simulink model "PMSMSC_FOC1_"  (R2021a)
settings: Solver=FixedStepDiscrete  StartTime=0.0  StopTime=25.0  FixedStep=1  RelTol=1e-3
undefined symbols (not defined in the file): DWORK0, DWORK1, DWORK2, sigbuilder_block, solver_time, speed_ki, speed_kp, Ts, Vd_ki, Vd_kp, Vdc, Vq_ki, Vq_kp
libraries: simulink x1
settings Model: DataDictionary=PMSMSC_FOC_datadictionary.sldd  Creator=comp  LastModifiedBy=LENOVO
settings SolverCC: AlgebraicLoopSolver=TrustRegion
settings OptimizationCC: DefaultParameterBehavior=Inlined  EnhancedBackFolding=on  PassReuseOutputArgsAs=Individual arguments  ZeroExternalMemoryAtStartup=off  ZeroInternalMemoryAtStartup=off  OptimizeBlockOrder=speed  DifferentSizesBufferReuse=on  OptimizationCustomize=off  EfficientTunableParamExpr=on
settings DebuggingCC: SignalInfNanChecking=error  ParameterPrecisionLossMsg=none  ParameterTunabilityLossMsg=error  UniqueDataStoreMsg=warning  SFMachineParentedDataDiag=warning
settings SFSimCC: MATLABDynamicMemAlloc=off  CustomCodeUndefinedFunction=UseInterfaceOnly
settings RTWCC: SystemTargetFile=ert.tlc  GenCodeOnly=on  TemplateMakefile=ert_default_tmf  GenerateReport=on  IncludeHyperlinkInReport=on  LaunchReport=on  GenerateTraceInfo=on  GenerateTraceReport=on  GenerateTraceReportSl=on
settings CodeAppCC: ForceParamTrailComments=on  IgnoreCustomStorageClasses=off  OperatorAnnotations=on  SimulinkDataObjDesc=on  SFDataObjDesc=on  InsertBlockDesc=on
settings ERTTargetCC: TargetLangStandard=C99 (ISO)  GenerateSampleERTMain=on  InlinedParameterPlacement=NonHierarchical  ERTCustomFileTemplate=example_file_process.tlc
settings ConfigComp: CovMetricSettings=dzw

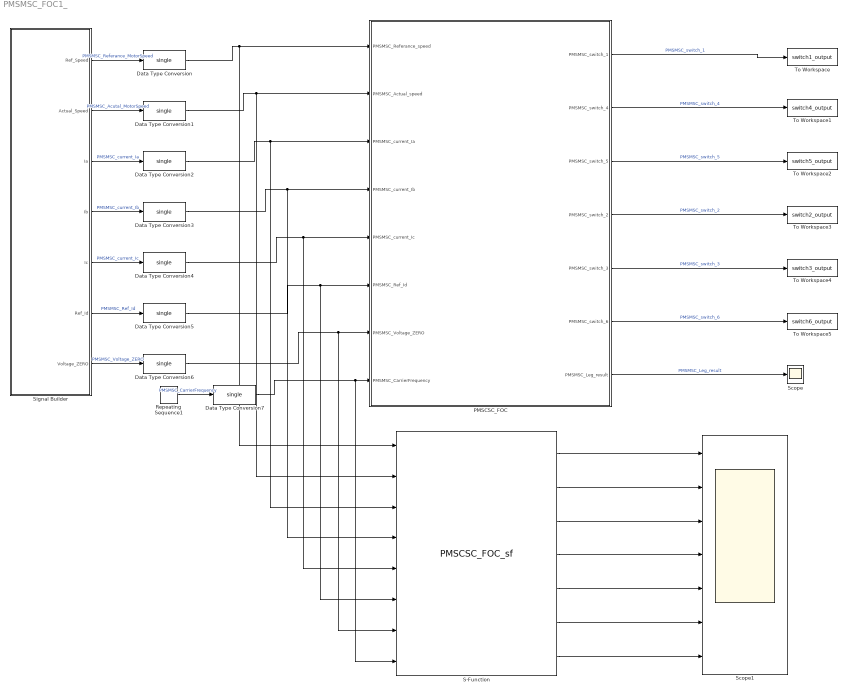
== system PMSMSC_FOC1_ ==
  Data Type Conversion{,1..7} (8 alike) : DataTypeConversion  OutDataTypeStr=single
  PMSCSC_FOC : Subsystem  TreatAsAtomicUnit=on
  Repeating Sequence1 : simulink/Sources/Repeating Sequence  rep_seq_t=[0 1]*[1/3000]  rep_seq_y=[0 0.02]
  S-Function : S-Function  FunctionName=PMSCSC_FOC_sf  SFunctionDeploymentMode=off  EnableBusSupport=off  SFcnStateName=DWORK0,DWORK1,DWORK2
      settings: SFcnIsStateOwnerBlock=on
  Scope : Scope
  Scope1 : Scope  NumInputPorts=7
  Signal Builder : Subsystem  Tag=STV Subsys  LoadFcn=sigbuilder_block('load');  StartFcn=sigbuilder_block('start');  StopFcn=sigbuilder_block('stop');  ClipboardFcn=sigbuilder_block('clipboard');  mask(Sigbuilder block){tuvar=[0:10]}
      mask help: Simulink:masks:SigbuilderBlock_MD
      mask init:
      | if ~strcmp(get_param(bdroot(gcbh),'SimulationStatus'),'stopped') tuvar = sigbuilder_block('maskInit'); end
      settings: CopyFcn=sigbuilder_block('copy');  DeleteFcn=sigbuilder_block('delete');  ModelCloseFcn=sigbuilder_block('modelClose');  PreSaveFcn=sigbuilder_block('preSave');  PauseFcn=sigbuilder_block('pause');  ContinueFcn=sigbuilder_block('continue');  NameChangeFcn=sigbuilder_block('namechange');  OpenFcn=sigbuilder_block('open',[6 30 1012.5 447.75 ]);  CloseFcn=sigbuilder_block('close');
      mask Display: plot(0, 0, 100, 100,[2, 2, 32, 32, 2], [68, 8, 8, 68, 68],[32, 2], [38, 38], [32, 19, 2],[53, 60, 44], [32, 17, 17, 2],[16, 16, 31, 31]);txt = getActiveGroup(gcbh);text(2, 100, txt,'verticalAlignment', 'top');
  To Workspace : ToWorkspace  VariableName=switch1_output  SaveFormat=Timeseries  SampleTime=-1
  To Workspace1 : ToWorkspace  VariableName=switch4_output  SaveFormat=Timeseries  SampleTime=-1
  To Workspace2 : ToWorkspace  VariableName=switch5_output  SaveFormat=Timeseries  SampleTime=-1
  To Workspace3 : ToWorkspace  VariableName=switch2_output  SaveFormat=Timeseries  SampleTime=-1
  To Workspace4 : ToWorkspace  VariableName=switch3_output  SaveFormat=Timeseries  SampleTime=-1
  To Workspace5 : ToWorkspace  VariableName=switch6_output  SaveFormat=Timeseries  SampleTime=-1
  wires:
  Signal Builder/3(Ia) -> Data Type Conversion2/1  "PMSMSC_current_Ia"
  PMSCSC_FOC/1(PMSMSC_switch_1) -> To Workspace/1  "PMSMSC_switch_1"
  PMSCSC_FOC/2(PMSMSC_switch_4) -> To Workspace1/1  "PMSMSC_switch_4"
  PMSCSC_FOC/3(PMSMSC_switch_5) -> To Workspace2/1  "PMSMSC_switch_5"
  PMSCSC_FOC/4(PMSMSC_switch_2) -> To Workspace3/1  "PMSMSC_switch_2"
  PMSCSC_FOC/6(PMSMSC_switch_6) -> To Workspace5/1  "PMSMSC_switch_6"
  PMSCSC_FOC/5(PMSMSC_switch_3) -> To Workspace4/1  "PMSMSC_switch_3"
  PMSCSC_FOC/7(PMSMSC_Leg_result) -> Scope/1  "PMSMSC_Leg_result"
  Repeating Sequence1/1 -> Data Type Conversion7/1  "PMSMSC_CarrierFrequency"
  Signal Builder/1(Ref_Speed) -> Data Type Conversion/1  "PMSMSC_Referance_MotorSpeed"
  Signal Builder/4(Ib) -> Data Type Conversion3/1  "PMSMSC_current_Ib"
  Signal Builder/7(Voltage_ZERO) -> Data Type Conversion6/1  "PMSMSC_Voltage_ZERO"
  Signal Builder/2(Actual_Speed) -> Data Type Conversion1/1  "PMSMSC_Acutal_MotorSpeed"
  Signal Builder/6(Ref_Id) -> Data Type Conversion5/1  "PMSMSC_Ref_Id"
  Signal Builder/5(Ic) -> Data Type Conversion4/1  "PMSMSC_current_Ic"
  Data Type Conversion/1 -> S-Function/1, PMSCSC_FOC/1(PMSMSC_Referance_speed)
  Data Type Conversion1/1 -> PMSCSC_FOC/2(PMSMSC_Actual_speed), S-Function/2
  Data Type Conversion2/1 -> PMSCSC_FOC/3(PMSMSC_current_Ia), S-Function/3
  Data Type Conversion3/1 -> PMSCSC_FOC/4(PMSMSC_current_Ib), S-Function/4
  Data Type Conversion4/1 -> PMSCSC_FOC/5(PMSMSC_current_Ic), S-Function/5
  Data Type Conversion5/1 -> PMSCSC_FOC/6(PMSMSC_Ref_Id), S-Function/6
  Data Type Conversion6/1 -> PMSCSC_FOC/7(PMSMSC_Voltage_ZERO), S-Function/7
  Data Type Conversion7/1 -> PMSCSC_FOC/8(PMSMSC_CarrierFrequency), S-Function/8
  S-Function/1 -> Scope1/1
  S-Function/2 -> Scope1/2
  S-Function/3 -> Scope1/3
  S-Function/4 -> Scope1/4
  S-Function/5 -> Scope1/5
  S-Function/6 -> Scope1/6
  S-Function/7 -> Scope1/7

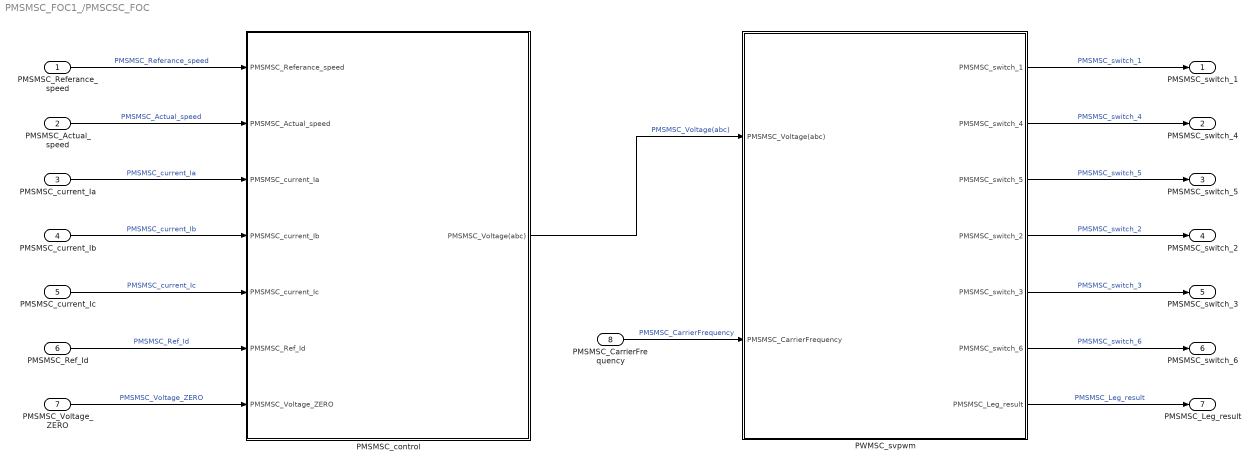
== system PMSMSC_FOC1_/PMSCSC_FOC ==
  PMSMSC_Referance_speed : Inport  OutDataTypeStr=single
  PMSMSC_Actual_speed : Inport  Port=2  OutDataTypeStr=single
  PMSMSC_current_Ia : Inport  Port=3  OutDataTypeStr=single
  PMSMSC_current_Ib : Inport  Port=4  OutDataTypeStr=single
  PMSMSC_current_Ic : Inport  Port=5  OutDataTypeStr=single
  PMSMSC_Ref_Id : Inport  Port=6  OutDataTypeStr=single
  PMSMSC_Voltage_ZERO : Inport  Port=7  OutDataTypeStr=single
  PMSMSC_CarrierFrequency : Inport  Port=8  OutDataTypeStr=single
  PMSMSC_control : Subsystem  TreatAsAtomicUnit=on
  PWMSC_svpwm : Subsystem  TreatAsAtomicUnit=on
  PMSMSC_switch_1 : Outport  OutDataTypeStr=single  VectorParamsAs1DForOutWhenUnconnected=off
  PMSMSC_switch_4 : Outport  Port=2  OutDataTypeStr=single  VectorParamsAs1DForOutWhenUnconnected=off
  PMSMSC_switch_5 : Outport  Port=3  OutDataTypeStr=single  VectorParamsAs1DForOutWhenUnconnected=off
  PMSMSC_switch_2 : Outport  Port=4  OutDataTypeStr=single  VectorParamsAs1DForOutWhenUnconnected=off
  PMSMSC_switch_3 : Outport  Port=5  OutDataTypeStr=single  VectorParamsAs1DForOutWhenUnconnected=off
  PMSMSC_switch_6 : Outport  Port=6  OutDataTypeStr=single  VectorParamsAs1DForOutWhenUnconnected=off
  PMSMSC_Leg_result : Outport  Port=7  OutDataTypeStr=single  VectorParamsAs1DForOutWhenUnconnected=off
  wires:
  PMSMSC_current_Ic/1 -> PMSMSC_control/5("PMSMSC_current_Ic ")  "PMSMSC_current_Ic"
  PMSMSC_Actual_speed/1 -> PMSMSC_control/2(PMSMSC_Actual_speed)  "PMSMSC_Actual_speed"
  PWMSC_svpwm/1(PMSMSC_switch_1) -> PMSMSC_switch_1/1  "PMSMSC_switch_1"
  PWMSC_svpwm/2(PMSMSC_switch_4) -> PMSMSC_switch_4/1  "PMSMSC_switch_4"
  PWMSC_svpwm/5(PMSMSC_switch_3) -> PMSMSC_switch_3/1  "PMSMSC_switch_3"
  PMSMSC_control/1(PMSMSC_Voltage(abc)) -> PWMSC_svpwm/1(PMSMSC_Voltage(abc))  "PMSMSC_Voltage(abc)"
  PWMSC_svpwm/3(PMSMSC_switch_5) -> PMSMSC_switch_5/1  "PMSMSC_switch_5"
  PWMSC_svpwm/4(PMSMSC_switch_2) -> PMSMSC_switch_2/1  "PMSMSC_switch_2"
  PMSMSC_Referance_speed/1 -> PMSMSC_control/1(PMSMSC_Referance_speed)  "PMSMSC_Referance_speed"
  PMSMSC_current_Ia/1 -> PMSMSC_control/3("PMSMSC_current_Ia ")  "PMSMSC_current_Ia"
  PMSMSC_current_Ib/1 -> PMSMSC_control/4("PMSMSC_current_Ib ")  "PMSMSC_current_Ib"
  PWMSC_svpwm/6(PMSMSC_switch_6) -> PMSMSC_switch_6/1  "PMSMSC_switch_6"
  PMSMSC_Ref_Id/1 -> PMSMSC_control/6("PMSMSC_Ref_Id ")  "PMSMSC_Ref_Id"
  PMSMSC_Voltage_ZERO/1 -> PMSMSC_control/7("PMSMSC_Voltage_ZERO ")  "PMSMSC_Voltage_ZERO"
  PWMSC_svpwm/7(PMSMSC_Leg_result) -> PMSMSC_Leg_result/1  "PMSMSC_Leg_result"
  PMSMSC_CarrierFrequency/1 -> PWMSC_svpwm/2(PMSMSC_CarrierFrequency)  "PMSMSC_CarrierFrequency"

== system PMSMSC_FOC1_/Signal Builder ==
  Demux : Demux  Tag=STV Demux  Outputs=7
      settings: DisplayOption=none
  FromWs : FromWorkspace  Tag=STV FromWs  VariableName=tuvar
      SigBuilderData=|
      | common.afterFinalStr = 'Extrapolate'
      | common.sampleTime = 0
      | dataSet.timeRange = [0 20]
      | dataSet.name = 'Sheet1'
      | sbobj.Name = 'Signal Builder'
      | sbobj.Groups.Name = 'Sheet1'
      | sbobj.Groups.Signals(1).Name = 'Ref_Speed'
      | sbobj.Groups.Signals(1).XData = [0 1 2 3 4 5 6 7 8 9 10 11 12 13 14 15 16 17 18 19 20]
      | sbobj.Groups.Signals(1).YData = [1200 1200 1200 1200 1200 1200 1200 1200 1200 1200 1200 1200 1200 1200 1200 1200 1200 1200 1200 1200 1200]
      | sbobj.Groups.Signals(2).Name = 'Actual_Speed'
      | sbobj.Groups.Signals(2).XData = [0 1 2 3 4 5 6 7 8 9 10 11 12 13 14 15 16 17 18 19 20]
      | sbobj.Groups.Signals(2).YData = [0 200 400 600 800 1000 1200 1400 1100 1150 1200 1250 1200 1280 1200 1270 1200 1260 1250 1200 1200]
      | sbobj.Groups.Signals(3).Name = 'Ia'
      | sbobj.Groups.Signals(3).XData = [0 1 2 3 4 5 6 7 8 9 10 11 12 13 14 15 16 17 18 19 20]
      | sbobj.Groups.Signals(3).YData = [0 10 20 30 40 50 60 50 60 60 60 60 60 60 60 60 60 60 60 60 60]
      | sbobj.Groups.Signals(4).Name = 'Ib'
      | sbobj.Groups.Signals(4).XData = [0 1 2 3 4 5 6 7 8 9 10 11 12 13 14 15 16 17 18 19 20]
      | sbobj.Groups.Signals(4).YData = [0 10 20 30 40 50 60 50 60 60 60 60 60 60 60 60 60 60 60 60 60]
      | sbobj.Groups.Signals(5).Name = 'Ic'
      | sbobj.Groups.Signals(5).XData = [0 1 2 3 4 5 6 7 8 9 10 11 12 13 14 15 16 17 18 19 20]
      | sbobj.Groups.Signals(5).YData = [0 10 20 30 40 50 60 50 60 60 60 60 60 60 60 60 60 60 60 60 60]
      | sbobj.Groups.Signals(6).Name = 'Ref_Id'
      | sbobj.Groups.Signals(6).XData = [0 1 2 3 4 5 6 7 8 9 10 11 12 13 14 15 16 17 18 19 20]
      | sbobj.Groups.Signals(6).YData = [0 0 0 0 0 0 0 0 0 0 0 0 0 0 0 0 0 0 0 0 0]
      | sbobj.Groups.Signals(7).Name = 'Voltage_ZERO'
      | sbobj.Groups.Signals(7).XData = [0 1 2 3 4 5 6 7 8 9 10 11 12 13 14 15 16 17 18 19 20]
      | sbobj.Groups.Signals(7).YData = [0 0 0 0 0 0 0 0 0 0 0 0 0 0 0 0 0 0 0 0 0]
      | sbobj.Groups.TimeRange = [0 20]
  Ref_Speed : Outport  Tag=STV Outport
  Actual_Speed : Outport  Tag=STV Outport  Port=2
  Ia : Outport  Tag=STV Outport  Port=3
  Ib : Outport  Tag=STV Outport  Port=4
  Ic : Outport  Tag=STV Outport  Port=5
  Ref_Id : Outport  Tag=STV Outport  Port=6
  Voltage_ZERO : Outport  Tag=STV Outport  Port=7
  wires:
  Demux/1 -> Ref_Speed/1
  FromWs/1 -> Demux/1
  Demux/2 -> Actual_Speed/1
  Demux/3 -> Ia/1
  Demux/4 -> Ib/1
  Demux/5 -> Ic/1
  Demux/6 -> Ref_Id/1
  Demux/7 -> Voltage_ZERO/1

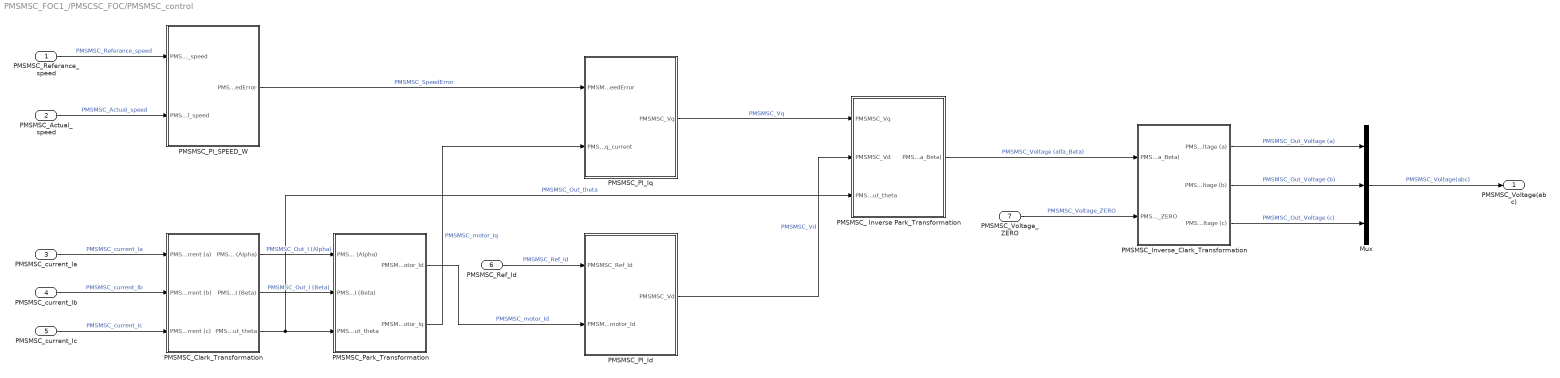
== system PMSMSC_FOC1_/PMSCSC_FOC/PMSMSC_control ==
  PMSMSC_Referance_speed : Inport  OutDataTypeStr=single
  PMSMSC_Actual_speed : Inport  Port=2  OutDataTypeStr=single
  "PMSMSC_current_Ia " : Inport  Port=3  OutDataTypeStr=single
  "PMSMSC_current_Ib " : Inport  Port=4  OutDataTypeStr=single
  "PMSMSC_current_Ic " : Inport  Port=5  OutDataTypeStr=single
  "PMSMSC_Ref_Id " : Inport  Port=6  OutDataTypeStr=single
  "PMSMSC_Voltage_ZERO " : Inport  Port=7  OutDataTypeStr=single
  Mux : Mux  Inputs=3
  PMSMSC_ Inverse Park_Transformation : Subsystem  TreatAsAtomicUnit=on
  "PMSMSC_Clark_Transformation " : Subsystem  TreatAsAtomicUnit=on
  PMSMSC_Inverse_Clark_Transformation : Subsystem  TreatAsAtomicUnit=on
  "PMSMSC_PI_Id " : Subsystem  TreatAsAtomicUnit=on
  "PMSMSC_PI_Iq " : Subsystem  TreatAsAtomicUnit=on
  "PMSMSC_PI_SPEED_W " : Subsystem  TreatAsAtomicUnit=on
  "PMSMSC_Park_Transformation " : Subsystem  TreatAsAtomicUnit=on
  PMSMSC_Voltage(abc) : Outport  OutDataTypeStr=single  VectorParamsAs1DForOutWhenUnconnected=off
  wires:
  PMSMSC_Inverse_Clark_Transformation/3("PMSMSC_Out_Voltage (c) ") -> Mux/3  "PMSMSC_Out_Voltage (c)"
  PMSMSC_Inverse_Clark_Transformation/1("PMSMSC_Out_Voltage (a) ") -> Mux/1  "PMSMSC_Out_Voltage (a)"
  PMSMSC_Actual_speed/1 -> "PMSMSC_PI_SPEED_W "/2(PMSMSC_Actual_speed)  "PMSMSC_Actual_speed"
  PMSMSC_Referance_speed/1 -> "PMSMSC_PI_SPEED_W "/1(PMSMSC_Referance_speed)  "PMSMSC_Referance_speed"
  "PMSMSC_Park_Transformation "/2(PMSMSC_motor_Iq) -> "PMSMSC_PI_Iq "/2(PMSMSC_Iq_current)  "PMSMSC_motor_Iq"
  "PMSMSC_Park_Transformation "/1("PMSMSC_motor_Id ") -> "PMSMSC_PI_Id "/2("PMSMSC_motor_Id ")  "PMSMSC_motor_Id"
  "PMSMSC_Ref_Id "/1 -> "PMSMSC_PI_Id "/1("PMSMSC_Ref_Id ")  "PMSMSC_Ref_Id"
  "PMSMSC_Clark_Transformation "/1(PMSMSC_Out_I (Alpha)) -> "PMSMSC_Park_Transformation "/1("PMSMSC_Out_I (Alpha) ")  "PMSMSC_Out_I (Alpha)"
  "PMSMSC_Clark_Transformation "/2(PMSMSC_Out_I (Beta)) -> "PMSMSC_Park_Transformation "/2("PMSMSC_Out_I (Beta) ")  "PMSMSC_Out_I (Beta)"
  "PMSMSC_PI_SPEED_W "/1(PMSMSC_SpeedError) -> "PMSMSC_PI_Iq "/1(PMSMSC_SpeedError)  "PMSMSC_SpeedError"
  "PMSMSC_PI_Id "/1("PMSMSC_Vd ") -> PMSMSC_ Inverse Park_Transformation/2("PMSMSC_Vd ")  "PMSMSC_Vd"
  "PMSMSC_PI_Iq "/1(PMSMSC_Vq) -> PMSMSC_ Inverse Park_Transformation/1("PMSMSC_Vq ")  "PMSMSC_Vq"
  "PMSMSC_Clark_Transformation "/3(PMSMSC_Out_theta) -> PMSMSC_ Inverse Park_Transformation/3("PMSMSC_Out_theta "), "PMSMSC_Park_Transformation "/3("PMSMSC_Out_theta ")  "PMSMSC_Out_theta"
  "PMSMSC_current_Ia "/1 -> "PMSMSC_Clark_Transformation "/1("PMSMSC_Inv_Out_Current (a) ")  "PMSMSC_current_Ia"
  "PMSMSC_current_Ib "/1 -> "PMSMSC_Clark_Transformation "/2("PMSMSC_Inv_Out_Current (b) ")  "PMSMSC_current_Ib"
  "PMSMSC_current_Ic "/1 -> "PMSMSC_Clark_Transformation "/3("PMSMSC_Inv_Out_Current (c) ")  "PMSMSC_current_Ic"
  Mux/1 -> PMSMSC_Voltage(abc)/1  "PMSMSC_Voltage(abc)"
  PMSMSC_Inverse_Clark_Transformation/2("PMSMSC_Out_Voltage (b) ") -> Mux/2  "PMSMSC_Out_Voltage (b)"
  PMSMSC_ Inverse Park_Transformation/1("PMSMSC_Voltage (alfa_Beta) ") -> PMSMSC_Inverse_Clark_Transformation/1(PMSMSC_Voltage (alfa_Beta))  "PMSMSC_Voltage (alfa_Beta)"
  "PMSMSC_Voltage_ZERO "/1 -> PMSMSC_Inverse_Clark_Transformation/2(PMSMSC_Voltage_ZERO)  "PMSMSC_Voltage_ZERO"

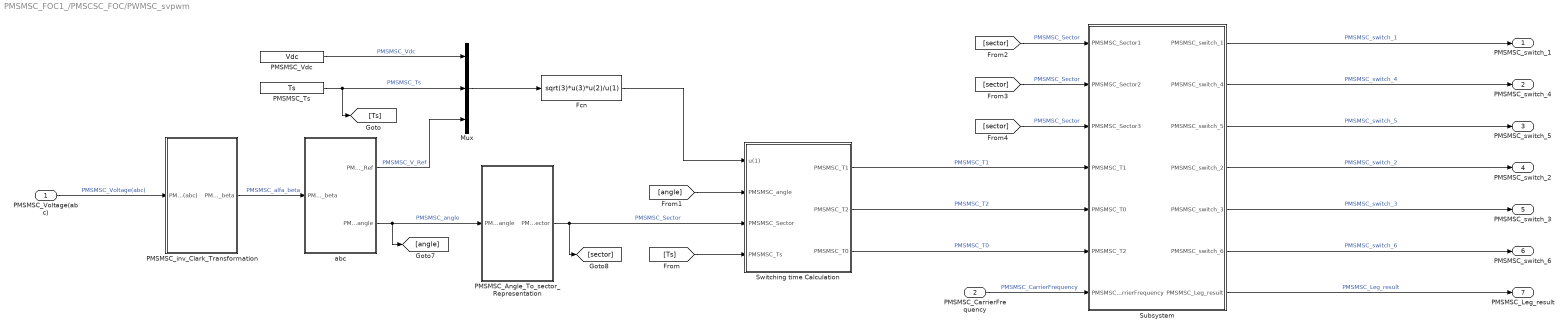
== system PMSMSC_FOC1_/PMSCSC_FOC/PWMSC_svpwm ==
  PMSMSC_Voltage(abc) : Inport  OutDataTypeStr=single
  PMSMSC_CarrierFrequency : Inport  Port=2  OutDataTypeStr=single
  Fcn : Fcn  Expr=sqrt(3)*u(3)*u(2)/u(1)
  Mux : Mux  Inputs=3
  PMSMSC_Angle_To_sector_Representation : Subsystem  TreatAsAtomicUnit=on
  PMSMSC_Ts : Constant  Value=Ts
  PMSMSC_Vdc : Constant  Value=Vdc
  PMSMSC_inv_Clark_Transformation : Subsystem  TreatAsAtomicUnit=on
  Subsystem : Subsystem  TreatAsAtomicUnit=on
  Switching time Calculation : Subsystem  TreatAsAtomicUnit=on
  abc : Subsystem  TreatAsAtomicUnit=on
  PMSMSC_switch_1 : Outport  OutDataTypeStr=single  VectorParamsAs1DForOutWhenUnconnected=off
  PMSMSC_switch_4 : Outport  Port=2  OutDataTypeStr=single  VectorParamsAs1DForOutWhenUnconnected=off
  PMSMSC_switch_5 : Outport  Port=3  OutDataTypeStr=single  VectorParamsAs1DForOutWhenUnconnected=off
  PMSMSC_switch_2 : Outport  Port=4  OutDataTypeStr=single  VectorParamsAs1DForOutWhenUnconnected=off
  PMSMSC_switch_3 : Outport  Port=5  OutDataTypeStr=single  VectorParamsAs1DForOutWhenUnconnected=off
  PMSMSC_switch_6 : Outport  Port=6  OutDataTypeStr=single  VectorParamsAs1DForOutWhenUnconnected=off
  PMSMSC_Leg_result : Outport  Port=7  OutDataTypeStr=single  VectorParamsAs1DForOutWhenUnconnected=off
  wires:
  abc/1(PMSMSC_V_Ref) -> Mux/3  "PMSMSC_V_Ref"
  PMSMSC_Vdc/1 -> Mux/1  "PMSMSC_Vdc"
  [Ts] -> Switching time Calculation/4(PMSMSC_Ts)
  [angle] -> Switching time Calculation/2(PMSMSC_angle)
  [sector] -> Subsystem/1(PMSMSC_Sector1)  "PMSMSC_Sector"
  Mux/1 -> Fcn/1
  abc/2("PMSMSC_angle ") -> [angle], PMSMSC_Angle_To_sector_Representation/1(PMSMSC_angle)  "PMSMSC_angle"
  Switching time Calculation/2(PMSMSC_T2) -> Subsystem/5(PMSMSC_T0)  "PMSMSC_T2"
  Subsystem/1(PMSMSC_switch_1) -> PMSMSC_switch_1/1  "PMSMSC_switch_1"
  [sector] -> Subsystem/3(PMSMSC_Sector3)  "PMSMSC_Sector"
  Fcn/1 -> Switching time Calculation/1(u(1))
  PMSMSC_Voltage(abc)/1 -> PMSMSC_inv_Clark_Transformation/1(PMSMSC_Voltage(abc))  "PMSMSC_Voltage(abc)"
  Switching time Calculation/1(PMSMSC_T1) -> Subsystem/4(PMSMSC_T1)  "PMSMSC_T1"
  PMSMSC_Angle_To_sector_Representation/1(PMSMSC_Sector) -> [sector], Switching time Calculation/3(PMSMSC_Sector)  "PMSMSC_Sector"
  PMSMSC_inv_Clark_Transformation/1(PMSMSC_alfa_beta) -> abc/1(PMSMSC_alfa_beta)  "PMSMSC_alfa_beta"
  PMSMSC_Ts/1 -> Mux/2, [Ts]  "PMSMSC_Ts"
  Subsystem/4(PMSMSC_switch_2) -> PMSMSC_switch_2/1  "PMSMSC_switch_2"
  Subsystem/3(PMSMSC_switch_5) -> PMSMSC_switch_5/1  "PMSMSC_switch_5"
  Switching time Calculation/3(PMSMSC_T0) -> Subsystem/6(PMSMSC_T2)  "PMSMSC_T0"
  [sector] -> Subsystem/2(PMSMSC_Sector2)  "PMSMSC_Sector"
  Subsystem/2(PMSMSC_switch_4) -> PMSMSC_switch_4/1  "PMSMSC_switch_4"
  Subsystem/6(PMSMSC_switch_6) -> PMSMSC_switch_6/1  "PMSMSC_switch_6"
  Subsystem/5(PMSMSC_switch_3) -> PMSMSC_switch_3/1  "PMSMSC_switch_3"
  Subsystem/7(PMSMSC_Leg_result) -> PMSMSC_Leg_result/1  "PMSMSC_Leg_result"
  PMSMSC_CarrierFrequency/1 -> Subsystem/7(PMSMSC_CarrierFrequency)  "PMSMSC_CarrierFrequency"

== system PMSMSC_FOC1_/PMSCSC_FOC/PMSMSC_control/PMSMSC_ Inverse Park_Transformation ==
  "PMSMSC_Vq " : Inport  OutDataTypeStr=single
  "PMSMSC_Vd " : Inport  Port=2  OutDataTypeStr=single
  "PMSMSC_Out_theta " : Inport  Port=3  OutDataTypeStr=single
  Mux : Mux  Inputs=3
  Mux1 : Mux  Inputs=2
  current_to_voltage_alfa : Fcn  Expr=u(1)*cos(u(3))-u(2)*sin(u(3))
  current_to_voltage_beta : Fcn  Expr=u(1)*sin(u(3))+u(2)*cos(u(3))
  "PMSMSC_Voltage (alfa_Beta) " : Outport  OutDataTypeStr=single  VectorParamsAs1DForOutWhenUnconnected=off
  wires:
  Mux1/1 -> "PMSMSC_Voltage (alfa_Beta) "/1  "PMSMSC_Voltage (alfa_Beta)"
  Mux/1 -> current_to_voltage_alfa/1, current_to_voltage_beta/1
  current_to_voltage_alfa/1 -> Mux1/1
  "PMSMSC_Vq "/1 -> Mux/1  "PMSMSC_Vq"
  "PMSMSC_Vd "/1 -> Mux/2  "PMSMSC_Vd"
  current_to_voltage_beta/1 -> Mux1/2
  "PMSMSC_Out_theta "/1 -> Mux/3  "PMSMSC_Out_theta"

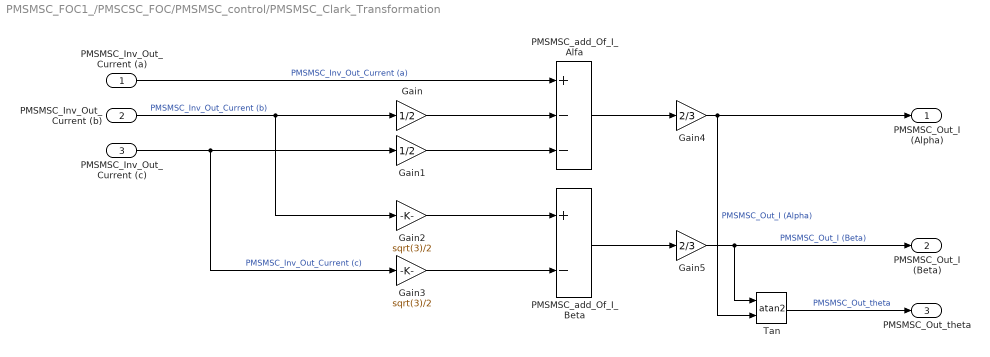
== system PMSMSC_FOC1_/PMSCSC_FOC/PMSMSC_control/PMSMSC_Clark_Transformation  ==
  "PMSMSC_Inv_Out_Current (a) " : Inport  OutDataTypeStr=single
  "PMSMSC_Inv_Out_Current (b) " : Inport  Port=2  OutDataTypeStr=single
  "PMSMSC_Inv_Out_Current (c) " : Inport  Port=3  OutDataTypeStr=single
  Gain : Gain  Gain=1/2  OutDataTypeStr=single
  Gain1 : Gain  Gain=1/2  OutDataTypeStr=single
  Gain2 : Gain  Gain=sqrt(3)/2  OutDataTypeStr=single
  Gain3 : Gain  Gain=sqrt(3)/2  OutDataTypeStr=single
  Gain4 : Gain  Gain=2/3  OutDataTypeStr=single
  Gain5 : Gain  Gain=2/3  OutDataTypeStr=single
  PMSMSC_add_Of_I_Alfa : Sum  Inputs=+--  AccumDataTypeStr=single
  PMSMSC_add_Of_I_Beta : Sum  Inputs=+-  AccumDataTypeStr=single
  Tan : Trigonometry  Operator=atan2
  PMSMSC_Out_I (Alpha) : Outport  OutDataTypeStr=single  VectorParamsAs1DForOutWhenUnconnected=off
  PMSMSC_Out_I (Beta) : Outport  Port=2  OutDataTypeStr=single  VectorParamsAs1DForOutWhenUnconnected=off
  PMSMSC_Out_theta : Outport  Port=3  OutDataTypeStr=single  VectorParamsAs1DForOutWhenUnconnected=off
  wires:
  Gain3/1 -> PMSMSC_add_Of_I_Beta/2
  "PMSMSC_Inv_Out_Current (b) "/1 -> Gain2/1, Gain/1  "PMSMSC_Inv_Out_Current (b)"
  Gain/1 -> PMSMSC_add_Of_I_Alfa/2
  Gain1/1 -> PMSMSC_add_Of_I_Alfa/3
  "PMSMSC_Inv_Out_Current (a) "/1 -> PMSMSC_add_Of_I_Alfa/1  "PMSMSC_Inv_Out_Current (a)"
  "PMSMSC_Inv_Out_Current (c) "/1 -> Gain3/1, Gain1/1  "PMSMSC_Inv_Out_Current (c)"
  PMSMSC_add_Of_I_Alfa/1 -> Gain4/1
  PMSMSC_add_Of_I_Beta/1 -> Gain5/1
  Gain2/1 -> PMSMSC_add_Of_I_Beta/1
  Gain5/1 -> Tan/1, PMSMSC_Out_I (Beta)/1  "PMSMSC_Out_I (Beta)"
  Gain4/1 -> Tan/2, PMSMSC_Out_I (Alpha)/1  "PMSMSC_Out_I (Alpha)"
  Tan/1 -> PMSMSC_Out_theta/1  "PMSMSC_Out_theta"

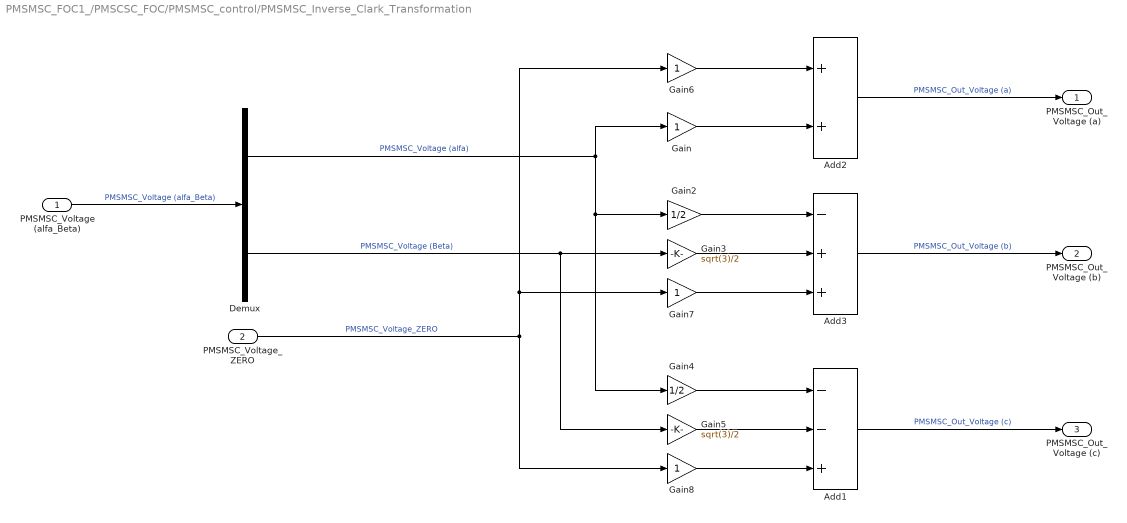
== system PMSMSC_FOC1_/PMSCSC_FOC/PMSMSC_control/PMSMSC_Inverse_Clark_Transformation ==
  PMSMSC_Voltage (alfa_Beta) : Inport  OutDataTypeStr=single
  PMSMSC_Voltage_ZERO : Inport  Port=2  OutDataTypeStr=single
  Add1 : Sum  Inputs=--+  AccumDataTypeStr=single
  Add2 : Sum  AccumDataTypeStr=single
  Add3 : Sum  Inputs=-++  AccumDataTypeStr=single
  Demux : Demux  Outputs=2
  Gain{,6..8} (4 alike) : Gain  OutDataTypeStr=single
  Gain2 : Gain  Gain=1/2  OutDataTypeStr=single
  Gain3 : Gain  Gain=sqrt(3)/2  OutDataTypeStr=single  SaturateOnIntegerOverflow=on
  Gain4 : Gain  Gain=1/2  OutDataTypeStr=single
  Gain5 : Gain  Gain=sqrt(3)/2  OutDataTypeStr=single
  "PMSMSC_Out_Voltage (a) " : Outport  OutDataTypeStr=single  VectorParamsAs1DForOutWhenUnconnected=off
  "PMSMSC_Out_Voltage (b) " : Outport  Port=2  OutDataTypeStr=single  VectorParamsAs1DForOutWhenUnconnected=off
  "PMSMSC_Out_Voltage (c) " : Outport  Port=3  OutDataTypeStr=single  VectorParamsAs1DForOutWhenUnconnected=off
  wires:
  Add3/1 -> "PMSMSC_Out_Voltage (b) "/1  "PMSMSC_Out_Voltage (b)"
  Add2/1 -> "PMSMSC_Out_Voltage (a) "/1  "PMSMSC_Out_Voltage (a)"
  Gain5/1 -> Add1/2
  Gain4/1 -> Add1/1
  Demux/2 -> Gain3/1, Gain5/1  "PMSMSC_Voltage (Beta)"
  Add1/1 -> "PMSMSC_Out_Voltage (c) "/1  "PMSMSC_Out_Voltage (c)"
  PMSMSC_Voltage_ZERO/1 -> Gain6/1, Gain7/1, Gain8/1  "PMSMSC_Voltage_ZERO"
  Demux/1 -> Gain/1, Gain2/1, Gain4/1  "PMSMSC_Voltage (alfa)"
  Gain3/1 -> Add3/2
  Gain8/1 -> Add1/3
  Gain2/1 -> Add3/1
  Gain6/1 -> Add2/1
  Gain/1 -> Add2/2
  Gain7/1 -> Add3/3
  PMSMSC_Voltage (alfa_Beta)/1 -> Demux/1  "PMSMSC_Voltage (alfa_Beta)"

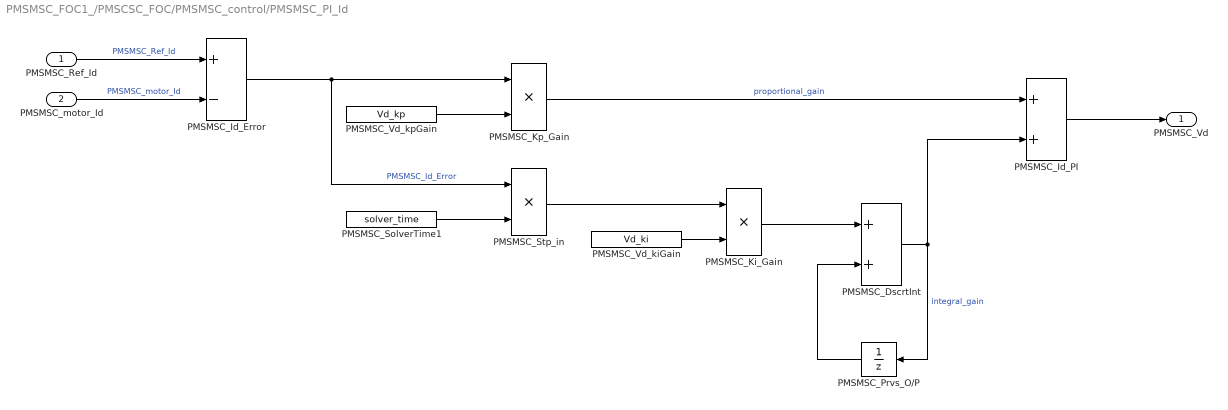
== system PMSMSC_FOC1_/PMSCSC_FOC/PMSMSC_control/PMSMSC_PI_Id  ==
  "PMSMSC_Ref_Id " : Inport  OutDataTypeStr=single
  "PMSMSC_motor_Id " : Inport  Port=2  OutDataTypeStr=single
  "PMSMSC_DscrtInt " : Sum  AccumDataTypeStr=single
  PMSMSC_Id_Error : Sum  Inputs=+-  AccumDataTypeStr=single
  PMSMSC_Id_PI : Sum  AccumDataTypeStr=single
  PMSMSC_Ki_Gain : Product  OutDataTypeStr=single
  PMSMSC_Kp_Gain : Product  OutDataTypeStr=single
  PMSMSC_Prvs_O/P : UnitDelay  SampleTime=-1  HasFrameUpgradeWarning=on
  PMSMSC_SolverTime1 : Constant  Value=solver_time
  "PMSMSC_Stp_in " : Product  OutDataTypeStr=single
  PMSMSC_Vd_kiGain : Constant  Value=Vd_ki
  PMSMSC_Vd_kpGain : Constant  Value=Vd_kp
  "PMSMSC_Vd " : Outport  OutDataTypeStr=single  VectorParamsAs1DForOutWhenUnconnected=off
  wires:
  PMSMSC_Kp_Gain/1 -> PMSMSC_Id_PI/1  "proportional_gain"
  PMSMSC_Vd_kiGain/1 -> PMSMSC_Ki_Gain/2
  PMSMSC_Ki_Gain/1 -> "PMSMSC_DscrtInt "/1
  PMSMSC_Vd_kpGain/1 -> PMSMSC_Kp_Gain/2
  PMSMSC_SolverTime1/1 -> "PMSMSC_Stp_in "/2
  "PMSMSC_motor_Id "/1 -> PMSMSC_Id_Error/2  "PMSMSC_motor_Id"
  PMSMSC_Id_PI/1 -> "PMSMSC_Vd "/1
  PMSMSC_Prvs_O/P/1 -> "PMSMSC_DscrtInt "/2
  PMSMSC_Id_Error/1 -> PMSMSC_Kp_Gain/1, "PMSMSC_Stp_in "/1  "PMSMSC_Id_Error"
  "PMSMSC_DscrtInt "/1 -> PMSMSC_Id_PI/2, PMSMSC_Prvs_O/P/1  "integral_gain"
  "PMSMSC_Ref_Id "/1 -> PMSMSC_Id_Error/1  "PMSMSC_Ref_Id"
  "PMSMSC_Stp_in "/1 -> PMSMSC_Ki_Gain/1

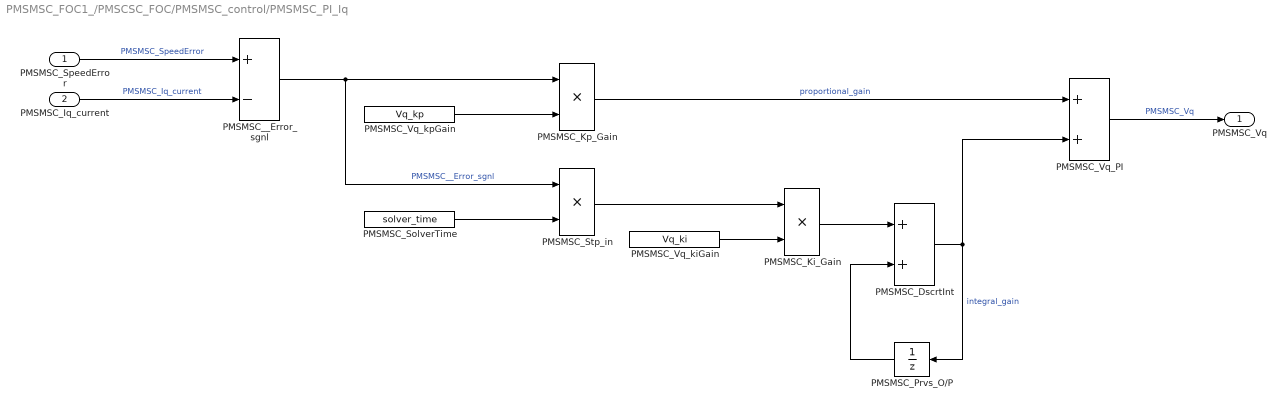
== system PMSMSC_FOC1_/PMSCSC_FOC/PMSMSC_control/PMSMSC_PI_Iq  ==
  PMSMSC_SpeedError : Inport  OutDataTypeStr=single
  PMSMSC_Iq_current : Inport  Port=2  OutDataTypeStr=single
  "PMSMSC_DscrtInt " : Sum  AccumDataTypeStr=single
  PMSMSC_Ki_Gain : Product  OutDataTypeStr=single
  PMSMSC_Kp_Gain : Product  OutDataTypeStr=single
  PMSMSC_Prvs_O/P : UnitDelay  SampleTime=-1  HasFrameUpgradeWarning=on
  PMSMSC_SolverTime : Constant  Value=solver_time
  "PMSMSC_Stp_in " : Product  OutDataTypeStr=single
  PMSMSC_Vq_PI : Sum  AccumDataTypeStr=single
  PMSMSC_Vq_kiGain : Constant  Value=Vq_ki
  PMSMSC_Vq_kpGain : Constant  Value=Vq_kp
  PMSMSC__Error_sgnl : Sum  Inputs=+-  AccumDataTypeStr=single
  PMSMSC_Vq : Outport  OutDataTypeStr=single  VectorParamsAs1DForOutWhenUnconnected=off
  wires:
  "PMSMSC_Stp_in "/1 -> PMSMSC_Ki_Gain/1
  PMSMSC_SpeedError/1 -> PMSMSC__Error_sgnl/1  "PMSMSC_SpeedError"
  "PMSMSC_DscrtInt "/1 -> PMSMSC_Vq_PI/2, PMSMSC_Prvs_O/P/1  "integral_gain"
  PMSMSC__Error_sgnl/1 -> "PMSMSC_Stp_in "/1, PMSMSC_Kp_Gain/1  "PMSMSC__Error_sgnl"
  PMSMSC_Prvs_O/P/1 -> "PMSMSC_DscrtInt "/2
  PMSMSC_Vq_PI/1 -> PMSMSC_Vq/1  "PMSMSC_Vq"
  PMSMSC_Iq_current/1 -> PMSMSC__Error_sgnl/2  "PMSMSC_Iq_current"
  PMSMSC_SolverTime/1 -> "PMSMSC_Stp_in "/2
  PMSMSC_Vq_kpGain/1 -> PMSMSC_Kp_Gain/2
  PMSMSC_Ki_Gain/1 -> "PMSMSC_DscrtInt "/1
  PMSMSC_Vq_kiGain/1 -> PMSMSC_Ki_Gain/2
  PMSMSC_Kp_Gain/1 -> PMSMSC_Vq_PI/1  "proportional_gain"

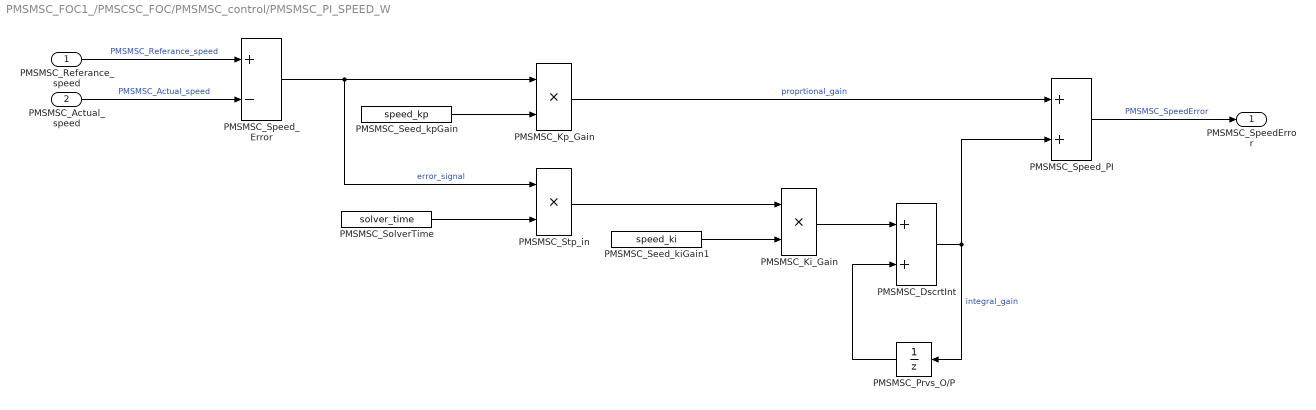
== system PMSMSC_FOC1_/PMSCSC_FOC/PMSMSC_control/PMSMSC_PI_SPEED_W  ==
  PMSMSC_Referance_speed : Inport  OutDataTypeStr=single
  PMSMSC_Actual_speed : Inport  Port=2  OutDataTypeStr=single
  "PMSMSC_DscrtInt " : Sum  AccumDataTypeStr=single
  PMSMSC_Ki_Gain : Product  OutDataTypeStr=single
  PMSMSC_Kp_Gain : Product  OutDataTypeStr=single
  PMSMSC_Prvs_O/P : UnitDelay  SampleTime=-1  HasFrameUpgradeWarning=on
  PMSMSC_Seed_kiGain1 : Constant  Value=speed_ki
  PMSMSC_Seed_kpGain : Constant  Value=speed_kp
  PMSMSC_SolverTime : Constant  Value=solver_time
  PMSMSC_Speed_Error : Sum  Inputs=+-  AccumDataTypeStr=single
  PMSMSC_Speed_PI : Sum  AccumDataTypeStr=single
  "PMSMSC_Stp_in " : Product  OutDataTypeStr=single
  PMSMSC_SpeedError : Outport  OutDataTypeStr=single  VectorParamsAs1DForOutWhenUnconnected=off
  wires:
  PMSMSC_Kp_Gain/1 -> PMSMSC_Speed_PI/1  "proprtional_gain"
  PMSMSC_Seed_kiGain1/1 -> PMSMSC_Ki_Gain/2
  PMSMSC_Ki_Gain/1 -> "PMSMSC_DscrtInt "/1
  PMSMSC_Seed_kpGain/1 -> PMSMSC_Kp_Gain/2
  PMSMSC_SolverTime/1 -> "PMSMSC_Stp_in "/2
  PMSMSC_Speed_PI/1 -> PMSMSC_SpeedError/1  "PMSMSC_SpeedError"
  PMSMSC_Prvs_O/P/1 -> "PMSMSC_DscrtInt "/2
  PMSMSC_Speed_Error/1 -> PMSMSC_Kp_Gain/1, "PMSMSC_Stp_in "/1  "error_signal"
  "PMSMSC_DscrtInt "/1 -> PMSMSC_Speed_PI/2, PMSMSC_Prvs_O/P/1  "integral_gain"
  PMSMSC_Referance_speed/1 -> PMSMSC_Speed_Error/1  "PMSMSC_Referance_speed"
  "PMSMSC_Stp_in "/1 -> PMSMSC_Ki_Gain/1
  PMSMSC_Actual_speed/1 -> PMSMSC_Speed_Error/2  "PMSMSC_Actual_speed"

== system PMSMSC_FOC1_/PMSCSC_FOC/PMSMSC_control/PMSMSC_Park_Transformation  ==
  "PMSMSC_Out_I (Alpha) " : Inport  OutDataTypeStr=single
  "PMSMSC_Out_I (Beta) " : Inport  Port=2  OutDataTypeStr=single
  "PMSMSC_Out_theta " : Inport  Port=3  OutDataTypeStr=single
  Fcn : Fcn  Expr=u(1)*cos(u(3))+u(2)*sin(u(3))
  Fcn1 : Fcn  Expr=-u(1)*sin(u(3))+u(2)*cos(u(3))
  Mux : Mux  Inputs=3
  "PMSMSC_motor_Id " : Outport  OutDataTypeStr=single  VectorParamsAs1DForOutWhenUnconnected=off
  PMSMSC_motor_Iq : Outport  Port=2  OutDataTypeStr=single  VectorParamsAs1DForOutWhenUnconnected=off
  wires:
  "PMSMSC_Out_I (Beta) "/1 -> Mux/2  "PMSMSC_Out_I (Beta)"
  "PMSMSC_Out_I (Alpha) "/1 -> Mux/1  "PMSMSC_Out_I (Alpha)"
  "PMSMSC_Out_theta "/1 -> Mux/3  "PMSMSC_Out_theta"
  Mux/1 -> Fcn1/1, Fcn/1
  Fcn/1 -> "PMSMSC_motor_Id "/1  "PMSMSC_motor_Id"
  Fcn1/1 -> PMSMSC_motor_Iq/1  "PMSMSC_motor_Iq"

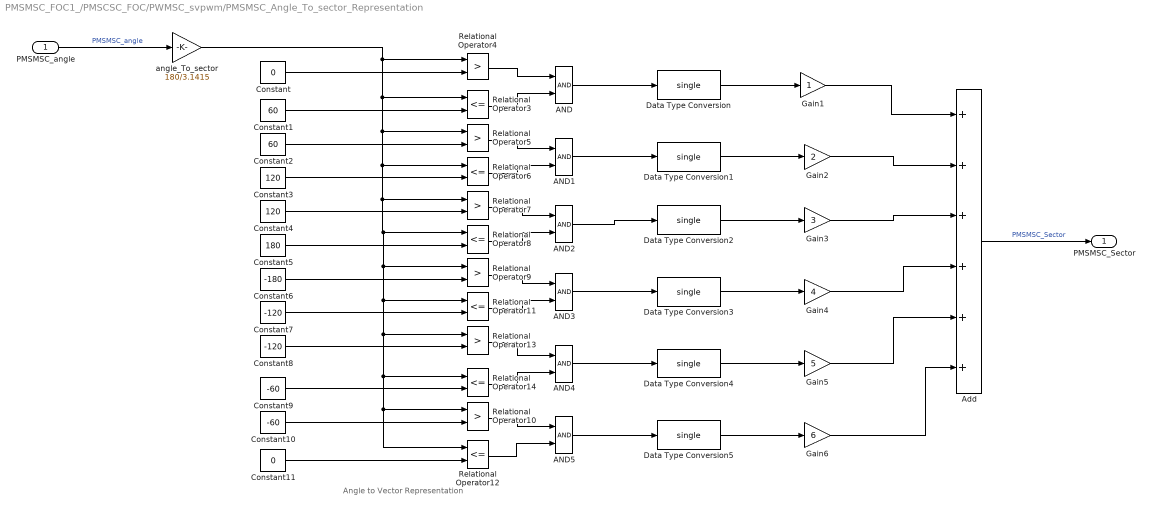
== system PMSMSC_FOC1_/PMSCSC_FOC/PWMSC_svpwm/PMSMSC_Angle_To_sector_Representation ==
  note: Angle to Vector Representation
  PMSMSC_angle : Inport  OutDataTypeStr=single
  AND{,1..5} (6 alike) : Logic  AllPortsSameDT=off  OutDataTypeStr=boolean
  Add : Sum  Inputs=++++++  AccumDataTypeStr=single
  Constant : Constant  Value=0  OutDataTypeStr=single
  Constant1 : Constant  Value=60  OutDataTypeStr=single
  Constant10 : Constant  Value=-60  OutDataTypeStr=single
  Constant11 : Constant  Value=0  OutDataTypeStr=single
  Constant2 : Constant  Value=60  OutDataTypeStr=single
  Constant3 : Constant  Value=120  OutDataTypeStr=single
  Constant4 : Constant  Value=120  OutDataTypeStr=single
  Constant5 : Constant  Value=180  OutDataTypeStr=single
  Constant6 : Constant  Value=-180  OutDataTypeStr=single
  Constant7 : Constant  Value=-120  OutDataTypeStr=single
  Constant8 : Constant  Value=-120  OutDataTypeStr=single
  Constant9 : Constant  Value=-60  OutDataTypeStr=single
  Data Type Conversion{,1..5} (6 alike) : DataTypeConversion  OutDataTypeStr=single
  Gain1 : Gain  OutDataTypeStr=single
  Gain2 : Gain  Gain=2  OutDataTypeStr=single
  Gain3 : Gain  Gain=3  OutDataTypeStr=single
  Gain4 : Gain  Gain=4  OutDataTypeStr=single
  Gain5 : Gain  Gain=5  OutDataTypeStr=single
  Gain6 : Gain  Gain=6  OutDataTypeStr=single
  Relational Operator{4..5,7,9..10,13} (6 alike) : RelationalOperator  Operator=>  OutDataTypeStr=boolean  RndMeth=Simplest
  Relational Operator{3,6,8,11..12,14} (6 alike) : RelationalOperator  Operator=<=  OutDataTypeStr=boolean  RndMeth=Simplest
  angle_To_sector : Gain  Gain=180/3.1415  OutDataTypeStr=single
  PMSMSC_Sector : Outport  OutDataTypeStr=single  VectorParamsAs1DForOutWhenUnconnected=off
  wires:
  Gain1/1 -> Add/1
  Data Type Conversion1/1 -> Gain2/1
  Constant1/1 -> Relational Operator3/2
  Data Type Conversion2/1 -> Gain3/1
  Add/1 -> PMSMSC_Sector/1  "PMSMSC_Sector"
  Relational Operator8/1 -> AND2/2
  Data Type Conversion/1 -> Gain1/1
  Constant5/1 -> Relational Operator8/2
  Gain3/1 -> Add/3
  Constant9/1 -> Relational Operator14/2
  angle_To_sector/1 -> Relational Operator14/1, Relational Operator12/1, Relational Operator10/1, Relational Operator13/1, Relational Operator11/1, Relational Operator9/1, Relational Operator8/1, Relational Operator7/1, Relational Operator6/1, Relational Operator5/1, Relational Operator3/1, Relational Operator4/1
  Data Type Conversion5/1 -> Gain6/1
  Constant11/1 -> Relational Operator12/2
  Constant4/1 -> Relational Operator7/2
  Data Type Conversion4/1 -> Gain5/1
  Constant/1 -> Relational Operator4/2
  Relational Operator3/1 -> AND/2
  AND/1 -> Data Type Conversion/1
  Relational Operator9/1 -> AND3/1
  Relational Operator7/1 -> AND2/1
  Data Type Conversion3/1 -> Gain4/1
  Relational Operator14/1 -> AND4/2
  Relational Operator6/1 -> AND1/2
  Constant7/1 -> Relational Operator11/2
  Constant10/1 -> Relational Operator10/2
  Relational Operator5/1 -> AND1/1
  Gain2/1 -> Add/2
  Gain4/1 -> Add/4
  Relational Operator13/1 -> AND4/1
  Constant2/1 -> Relational Operator5/2
  Constant3/1 -> Relational Operator6/2
  Relational Operator12/1 -> AND5/2
  Relational Operator4/1 -> AND/1
  Gain5/1 -> Add/5
  AND1/1 -> Data Type Conversion1/1
  Constant6/1 -> Relational Operator9/2
  AND5/1 -> Data Type Conversion5/1
  AND2/1 -> Data Type Conversion2/1
  Relational Operator10/1 -> AND5/1
  Relational Operator11/1 -> AND3/2
  AND4/1 -> Data Type Conversion4/1
  Constant8/1 -> Relational Operator13/2
  AND3/1 -> Data Type Conversion3/1
  Gain6/1 -> Add/6
  PMSMSC_angle/1 -> angle_To_sector/1  "PMSMSC_angle"

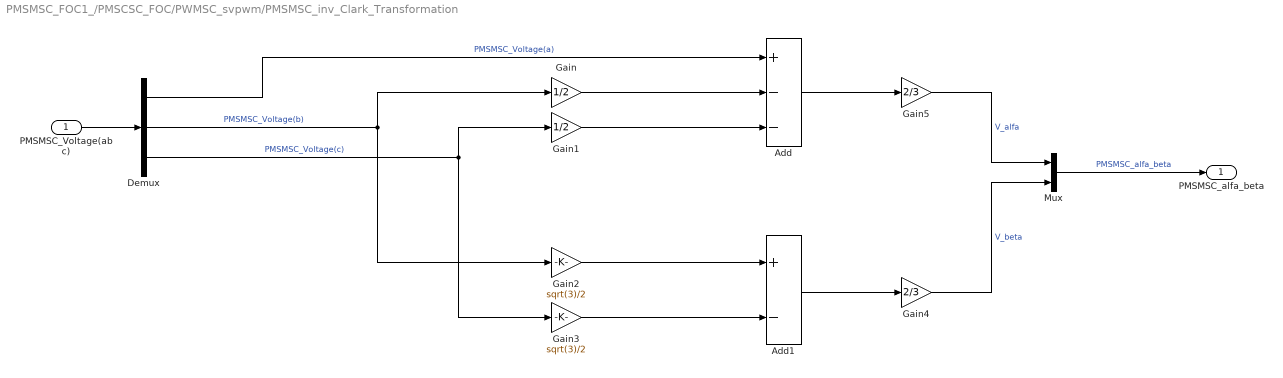
== system PMSMSC_FOC1_/PMSCSC_FOC/PWMSC_svpwm/PMSMSC_inv_Clark_Transformation ==
  PMSMSC_Voltage(abc) : Inport  OutDataTypeStr=single
  Add : Sum  Inputs=+--  AccumDataTypeStr=single
  Add1 : Sum  Inputs=+-  AccumDataTypeStr=single
  Demux : Demux  Outputs=3
  Gain : Gain  Gain=1/2  OutDataTypeStr=single
  Gain1 : Gain  Gain=1/2  OutDataTypeStr=single
  Gain2 : Gain  Gain=sqrt(3)/2  OutDataTypeStr=single
  Gain3 : Gain  Gain=sqrt(3)/2  OutDataTypeStr=single
  Gain4 : Gain  Gain=2/3  OutDataTypeStr=single
  Gain5 : Gain  Gain=2/3  OutDataTypeStr=single
  Mux : Mux  Inputs=2
  PMSMSC_alfa_beta : Outport  OutDataTypeStr=single  VectorParamsAs1DForOutWhenUnconnected=off
  wires:
  Demux/2 -> Gain2/1, Gain/1  "PMSMSC_Voltage(b)"
  Demux/1 -> Add/1  "PMSMSC_Voltage(a)"
  Add1/1 -> Gain4/1
  Add/1 -> Gain5/1
  Demux/3 -> Gain3/1, Gain1/1  "PMSMSC_Voltage(c)"
  Gain2/1 -> Add1/1
  Gain/1 -> Add/2
  Gain3/1 -> Add1/2
  Gain1/1 -> Add/3
  PMSMSC_Voltage(abc)/1 -> Demux/1
  Gain5/1 -> Mux/1  "V_alfa"
  Gain4/1 -> Mux/2  "V_beta"
  Mux/1 -> PMSMSC_alfa_beta/1  "PMSMSC_alfa_beta"

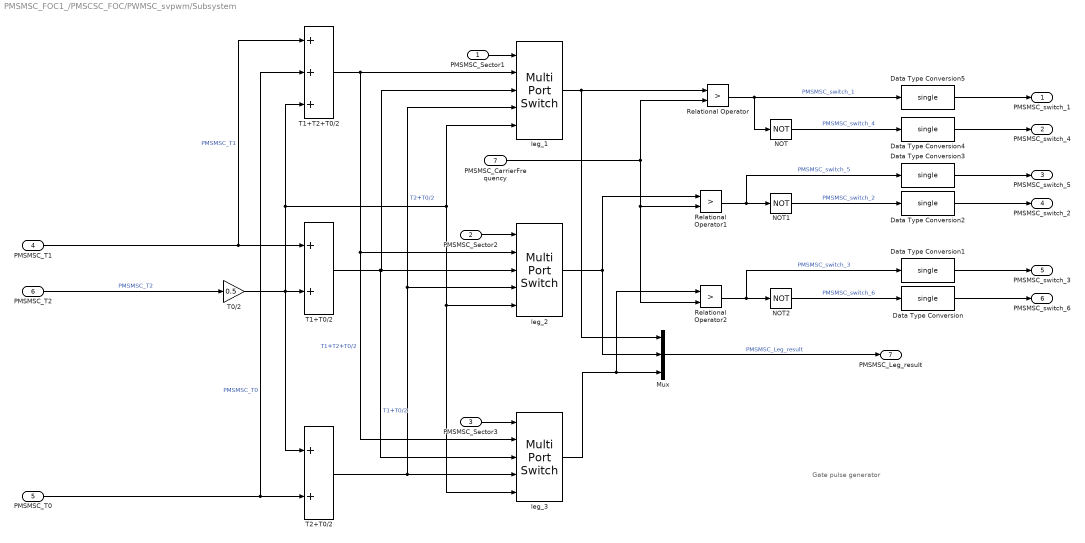
== system PMSMSC_FOC1_/PMSCSC_FOC/PWMSC_svpwm/Subsystem ==
  note: Gate pulse generator
  PMSMSC_Sector1 : Inport  OutDataTypeStr=single
  PMSMSC_Sector2 : Inport  Port=2  OutDataTypeStr=single
  PMSMSC_Sector3 : Inport  Port=3  OutDataTypeStr=single
  PMSMSC_T1 : Inport  Port=4  OutDataTypeStr=single
  PMSMSC_T0 : Inport  Port=5  OutDataTypeStr=single
  PMSMSC_T2 : Inport  Port=6  OutDataTypeStr=single
  PMSMSC_CarrierFrequency : Inport  Port=7  OutDataTypeStr=single
  Data Type Conversion{,1..5} (6 alike) : DataTypeConversion  OutDataTypeStr=single
  Mux : Mux  Inputs=3
  NOT : Logic  Operator=NOT  AllPortsSameDT=off  OutDataTypeStr=boolean
  NOT1 : Logic  Operator=NOT  AllPortsSameDT=off  OutDataTypeStr=boolean
  NOT2 : Logic  Operator=NOT  AllPortsSameDT=off  OutDataTypeStr=boolean
  Relational Operator : RelationalOperator  Operator=>  OutDataTypeStr=boolean  RndMeth=Simplest
  Relational Operator1 : RelationalOperator  Operator=>  OutDataTypeStr=boolean  RndMeth=Simplest
  Relational Operator2 : RelationalOperator  Operator=>  OutDataTypeStr=boolean  RndMeth=Simplest
  T0/2 : Gain  Gain=0.5  OutDataTypeStr=single
  T1+T0/2 : Sum  AccumDataTypeStr=single
  T1+T2+T0/2 : Sum  Inputs=+++  AccumDataTypeStr=single
  T2+T0/2 : Sum  AccumDataTypeStr=single
  "leg_1 " : MultiPortSwitch  DataPortOrder=Specify indices  DataPortIndices={[1,6],2,5,[3,4]}  DiagnosticForDefault=None  OutDataTypeStr=single
  "leg_2 " : MultiPortSwitch  DataPortOrder=Specify indices  DataPortIndices={[2,3],4,1,[5,6]}  DiagnosticForDefault=None  OutDataTypeStr=single
  "leg_3 " : MultiPortSwitch  DataPortOrder=Specify indices  DataPortIndices={[4,5],6,3,[1,2]}  DiagnosticForDefault=None  OutDataTypeStr=single
  PMSMSC_switch_1 : Outport  OutDataTypeStr=single  VectorParamsAs1DForOutWhenUnconnected=off
  PMSMSC_switch_4 : Outport  Port=2  OutDataTypeStr=single  VectorParamsAs1DForOutWhenUnconnected=off
  PMSMSC_switch_5 : Outport  Port=3  OutDataTypeStr=single  VectorParamsAs1DForOutWhenUnconnected=off
  PMSMSC_switch_2 : Outport  Port=4  OutDataTypeStr=single  VectorParamsAs1DForOutWhenUnconnected=off
  PMSMSC_switch_3 : Outport  Port=5  OutDataTypeStr=single  VectorParamsAs1DForOutWhenUnconnected=off
  PMSMSC_switch_6 : Outport  Port=6  OutDataTypeStr=single  VectorParamsAs1DForOutWhenUnconnected=off
  PMSMSC_Leg_result : Outport  Port=7  OutDataTypeStr=single  VectorParamsAs1DForOutWhenUnconnected=off
  wires:
  PMSMSC_CarrierFrequency/1 -> Relational Operator2/2, Relational Operator1/2, Relational Operator/2
  Relational Operator1/1 -> Data Type Conversion3/1, NOT1/1  "PMSMSC_switch_5"
  Relational Operator2/1 -> Data Type Conversion1/1, NOT2/1  "PMSMSC_switch_3"
  T1+T2+T0/2/1 -> "leg_3 "/2, "leg_2 "/2, "leg_1 "/2  "T1+T2+T0/2"
  PMSMSC_Sector2/1 -> "leg_2 "/1
  T2+T0/2/1 -> "leg_1 "/4, "leg_2 "/4, "leg_3 "/4  "T2+T0/2"
  T0/2/1 -> T2+T0/2/1, T1+T0/2/2, "leg_3 "/5, "leg_2 "/5, "leg_1 "/5, T1+T2+T0/2/3
  "leg_3 "/1 -> Relational Operator2/1, Mux/3
  "leg_2 "/1 -> Mux/2, Relational Operator1/1
  PMSMSC_T0/1 -> T1+T2+T0/2/2, T2+T0/2/2  "PMSMSC_T0"
  PMSMSC_Sector3/1 -> "leg_3 "/1
  PMSMSC_T1/1 -> T1+T2+T0/2/1, T1+T0/2/1  "PMSMSC_T1"
  "leg_1 "/1 -> Mux/1, Relational Operator/1
  PMSMSC_Sector1/1 -> "leg_1 "/1
  T1+T0/2/1 -> "leg_3 "/3, "leg_1 "/3, "leg_2 "/3  "T1+T0/2"
  NOT1/1 -> Data Type Conversion2/1  "PMSMSC_switch_2"
  Relational Operator/1 -> Data Type Conversion5/1, NOT/1  "PMSMSC_switch_1"
  NOT2/1 -> Data Type Conversion/1  "PMSMSC_switch_6"
  PMSMSC_T2/1 -> T0/2/1  "PMSMSC_T2"
  Mux/1 -> PMSMSC_Leg_result/1  "PMSMSC_Leg_result"
  NOT/1 -> Data Type Conversion4/1  "PMSMSC_switch_4"
  Data Type Conversion/1 -> PMSMSC_switch_6/1
  Data Type Conversion1/1 -> PMSMSC_switch_3/1
  Data Type Conversion2/1 -> PMSMSC_switch_2/1
  Data Type Conversion3/1 -> PMSMSC_switch_5/1
  Data Type Conversion4/1 -> PMSMSC_switch_4/1
  Data Type Conversion5/1 -> PMSMSC_switch_1/1

== system PMSMSC_FOC1_/PMSCSC_FOC/PWMSC_svpwm/Switching time Calculation ==
  u(1) : Inport  OutDataTypeStr=single
  PMSMSC_angle : Inport  Port=2  OutDataTypeStr=single
  PMSMSC_Sector : Inport  Port=3  OutDataTypeStr=single
  PMSMSC_Ts : Inport  Port=4  OutDataTypeStr=single
  Mux : Mux  Inputs=3
  TS-T1-T2 : Sum  Inputs=+--  AccumDataTypeStr=single
  T_1 : Fcn  Expr=u(1)*sin(u(3)*pi/3-u(2))
  T_2 : Fcn  Expr=u(1)*sin(-(u(3)-1)*pi/3+u(2))
  PMSMSC_T1 : Outport  OutDataTypeStr=single
  PMSMSC_T2 : Outport  Port=2  OutDataTypeStr=single
  PMSMSC_T0 : Outport  Port=3  OutDataTypeStr=single
  wires:
  u(1)/1 -> Mux/1
  T_1/1 -> PMSMSC_T1/1, TS-T1-T2/2  "PMSMSC_T1"
  PMSMSC_Ts/1 -> TS-T1-T2/1  "PMSMSC_Ts"
  T_2/1 -> PMSMSC_T2/1, TS-T1-T2/3  "PMSMSC_T2"
  Mux/1 -> T_2/1, T_1/1
  TS-T1-T2/1 -> PMSMSC_T0/1  "PMSMSC_T0"
  PMSMSC_angle/1 -> Mux/2  "PMSMSC_angle"
  PMSMSC_Sector/1 -> Mux/3  "PMSMSC_Sector"

== system PMSMSC_FOC1_/PMSCSC_FOC/PWMSC_svpwm/abc ==
  PMSMSC_alfa_beta : Inport  OutDataTypeStr=single
  Add : Sum  AccumDataTypeStr=single
  Demux : Demux  Outputs=2
  Square : Math  Operator=square  SignedPower=on  OutDataTypeStr=single  SaturateOnIntegerOverflow=on
  Square Root : Sqrt  OutDataTypeStr=single  IntermediateResultsDataTypeStr=single  SaturateOnIntegerOverflow=on
  Square1 : Math  Operator=square  SignedPower=on  OutDataTypeStr=single  SaturateOnIntegerOverflow=on
  Tan : Trigonometry  Operator=atan2
  PMSMSC_V_Ref : Outport  OutDataTypeStr=single  VectorParamsAs1DForOutWhenUnconnected=off
  "PMSMSC_angle " : Outport  Port=2  OutDataTypeStr=single  VectorParamsAs1DForOutWhenUnconnected=off
  wires:
  Demux/1 -> Tan/1, Square/1
  Demux/2 -> Tan/2, Square1/1
  Square/1 -> Add/1
  Square1/1 -> Add/2
  Add/1 -> Square Root/1
  Square Root/1 -> PMSMSC_V_Ref/1  "PMSMSC_V_Ref"
  PMSMSC_alfa_beta/1 -> Demux/1  "PMSMSC_alfa_beta"
  Tan/1 -> "PMSMSC_angle "/1  "PMSMSC_angle"
